simulink library "Pressure_Drop_StorageHX"  (Simulink 8.2)
settings: Solver=ode45  StartTime=0.0  StopTime=10.0  RelTol=1e-3
undefined symbols (not defined in the file): dia, hgt
libraries: carnot x3
settings Model: Creator=drhf  LastModifiedBy=drhf

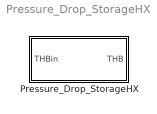
== system Pressure_Drop_StorageHX ==
  Pressure_Drop_StorageHX : Subsystem  mask(Pressure drop of tube heat exchanger in a storage){dia=dia, hgt=hgt}
      mask prompts: dia "Diameter in m"; hgt "height difference inlet-outlet"
      mask help:
      | Calculates the pressure drop in a tube heat exchanger according to:
      | dp = qua*mdot^2 + lin*mdot + density*grav*height
      mask Help: web(fullfile(path_carnot('help'),'Pressure_Drop_StorageHX.html'),'-helpbrowser')

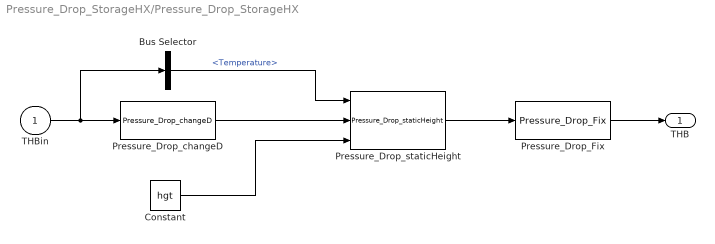
== system Pressure_Drop_StorageHX/Pressure_Drop_StorageHX ==
  THBin : Inport
  Bus Selector : BusSelector  OutputSignals=Temperature
  Constant : Constant  Value=hgt
  Pressure_Drop_Fix : carnot/Basic/Pressure_Drop/Pressure_Drop_Fix  con=0  lin=dplin  qua=dpqua
  Pressure_Drop_changeD : carnot/Basic/Pressure_Drop/Pressure_Drop_changeD  dia=dia
  Pressure_Drop_staticHeight : carnot/Basic/Pressure_Drop/Pressure_Drop_staticHeight
  THB : Outport
  wires:
  Pressure_Drop_Fix/1 -> THB/1
  Bus Selector/1 -> Pressure_Drop_staticHeight/1  "<Temperature>"
  THBin/1 -> Bus Selector/1, Pressure_Drop_changeD/1
  Constant/1 -> Pressure_Drop_staticHeight/3
  Pressure_Drop_changeD/1 -> Pressure_Drop_staticHeight/2
  Pressure_Drop_staticHeight/1 -> Pressure_Drop_Fix/1
